simulink library "Thermohydraulic"  (R2017a)
settings: Solver=ode45  StartTime=0.0  StopTime=10.0  RelTol=1e-3  EnableMultiTasking=on
undefined symbols (not defined in the file): CI, DiscIntNeverNeededParam, h, m, m3
settings Model: Creator=jpp  LastModifiedBy=La de Marcelo
settings DataIOCC: LimitDataPoints=on  SaveFormat=Array
settings OptimizationCC: DefaultParameterBehavior=Inlined  ExpressionDepthLimit=2147483647  LifeSpan=inf
settings DebuggingCC: UnderspecifiedInitializationDetection=Classic  MergeDetectMultiDrivingBlocksExec=none  SolverPrmCheckMsg=warning  StateNameClashWarn=warning  SFUnexpectedBacktrackingDiag=warning  SFNoUnconditionalDefaultTransitionDiag=warning  SFExecutionAtInitializationDiag=none
settings HardwareCC: ProdBitPerPointer=32  ProdBitPerSizeT=32  ProdBitPerPtrDiffT=32  ProdLargestAtomicFloat=None  ProdIntDivRoundTo=Undefined  ProdEndianess=Unspecified  ProdWordSize=32  ProdHWDeviceType=32-bit Generic
settings ModelReferenceCC: PropagateSignalLabelsOutOfModel=off
settings GRTTargetCC: TargetLangStandard=C89/C90 (ANSI)  GeneratePreprocessorConditionals=Disable all
settings ConfigComp: CovMetricSettings=dw  CovHtmlReporting=on  CovSaveCumulativeToWorkspaceVar=on  CovSaveSingleToWorkspaceVar=on  CovExternalEMLEnable=off

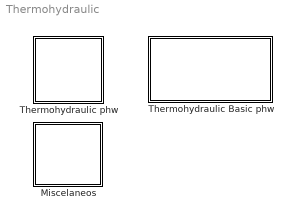
== system Thermohydraulic ==
  Miscelaneos : Subsystem
  Thermohydraulic Basic phw : Subsystem
      settings: OpenFcn=ThermohydraulicBasic_phw
  Thermohydraulic phw : Subsystem
      settings: OpenFcn=th_phw

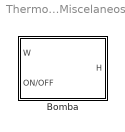
== system Thermohydraulic/Miscelaneos ==
  Bomba : Subsystem  mask{curvaQH_Q=[0.0 100.0 200.0 250.0 300.0 350.0] %(m3/h), curvaQH_H=[32.0 31.6 31.0 30.5 29.0 27.0] %(m), Tao=1.0, Ts=0.25, Descripcion=Curva Caracteristica Bomba}
      mask prompts: Tao "Tao (tss=5Tao)"; Ts "Tiempo Muestreo"
      mask DialogControl DescGroupVar Prompt: Modelo Básico de Bomba
      mask DialogControl DescTextVar Prompt: Cuenta con curva Q-H e inercia.
      mask DialogControl ParameterGroupVar Prompt: Parametros Modelado

== system Thermohydraulic/Thermohydraulic Basic phw ==

== system Thermohydraulic/Thermohydraulic phw ==

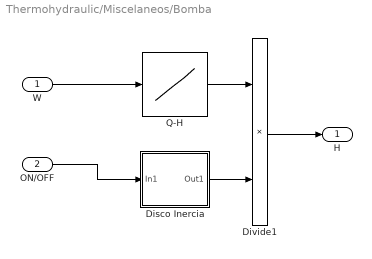
== system Thermohydraulic/Miscelaneos/Bomba ==
  W : Inport
  ON/OFF : Inport  Port=2
  Disco Inercia : Subsystem
  Divide1 : Product  Inputs=**
  Q-H : Lookup_n-D  NumberOfTableDimensions=1  BreakpointsForDimension1=curvaQH_Q  Table=curvaQH_H  RndMeth=Simplest  InputSameDT=on
  H : Outport
  wires:
  Q-H/1 -> Divide1/1
  W/1 -> Q-H/1
  ON/OFF/1 -> Disco Inercia/1(In1)
  Divide1/1 -> H/1
  Disco Inercia/1(Out1) -> Divide1/2

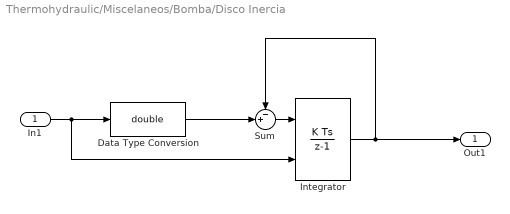
== system Thermohydraulic/Miscelaneos/Bomba/Disco Inercia ==
  In1 : Inport
  Data Type Conversion : DataTypeConversion  OutDataTypeStr=double
  Integrator : DiscreteIntegrator  gainval=Tao  InitialConditionSource=external  InitialCondition=CI  InitialConditionSetting=State (most efficient)  SampleTime=Ts  ICPrevOutput=DiscIntNeverNeededParam  ICPrevScaledInput=DiscIntNeverNeededParam
  Sum : Sum  Inputs=-+|
  Out1 : Outport
  wires:
  Integrator/1 -> Sum/1, Out1/1
  Sum/1 -> Integrator/1
  Data Type Conversion/1 -> Sum/2
  In1/1 -> Integrator/2, Data Type Conversion/1
